simulink model "wb_try2"  (R2016b)
settings: Solver=FixedStepDiscrete  StartTime=0.0  StopTime=99/paramRadarMT.prf  RelTol=1e-3  EnableMultiTasking=on
PreLoadFcn:
  | helperslexMonostaticRadarMultipleTargetsParam()
undefined symbols (not defined in the file or in its folder): paramRadarMT, phased, physconst
libraries: phasedenvlib x5, phasedtxrxlib x4, phaseddetectlib x3, phasedwavlib x2, simulink x1, phasedbflib x1
CloseFcn:
  | clear paramRadarMT
Description:
  | Monostatic Radar with Three Targets
settings Model: Creator=The MathWorks, Inc.  LastModifiedBy=CHAITRA
settings DataIOCC: LimitDataPoints=on  SaveFormat=Array  SaveOutput=off  SaveTime=off
settings OptimizationCC: ExpressionDepthLimit=2147483647  LifeSpan=inf
settings DebuggingCC: ReadBeforeWriteMsg=DisableAll  WriteAfterWriteMsg=DisableAll  WriteAfterReadMsg=DisableAll  UnderspecifiedInitializationDetection=Classic  MergeDetectMultiDrivingBlocksExec=none  SolverPrmCheckMsg=warning  InheritedTsInSrcMsg=none  MultiTaskDSMMsg=none  FcnCallInpInsideContextMsg=warning  AllowSymbolicDim=off  StateNameClashWarn=warning  SFUnexpectedBacktrackingDiag=warning  SFNoUnconditionalDefaultTransitionDiag=warning  SFExecutionAtInitializationDiag=none
settings HardwareCC: ProdBitPerPointer=32  ProdBitPerSizeT=32  ProdBitPerPtrDiffT=32  ProdLargestAtomicFloat=None  ProdIntDivRoundTo=Undefined  ProdEndianess=Unspecified  ProdWordSize=32  ProdHWDeviceType=32-bit Generic
settings ModelReferenceCC: UpdateModelReferenceTargets=IfOutOfDate  PropagateSignalLabelsOutOfModel=off
settings SFSimCC: SFSimEcho=off  SimParseCustomCode=off
settings GRTTargetCC: TargetLangStandard=C89/C90 (ANSI)  GeneratePreprocessorConditionals=Disable all  CombineOutputUpdateFcns=off  GRTInterface=on
settings ConfigComp: CovMetricSettings=dw  CovHtmlReporting=on  CovSaveCumulativeToWorkspaceVar=on  CovSaveSingleToWorkspaceVar=on  CovExternalEMLEnable=off  CovSFcnEnable=off

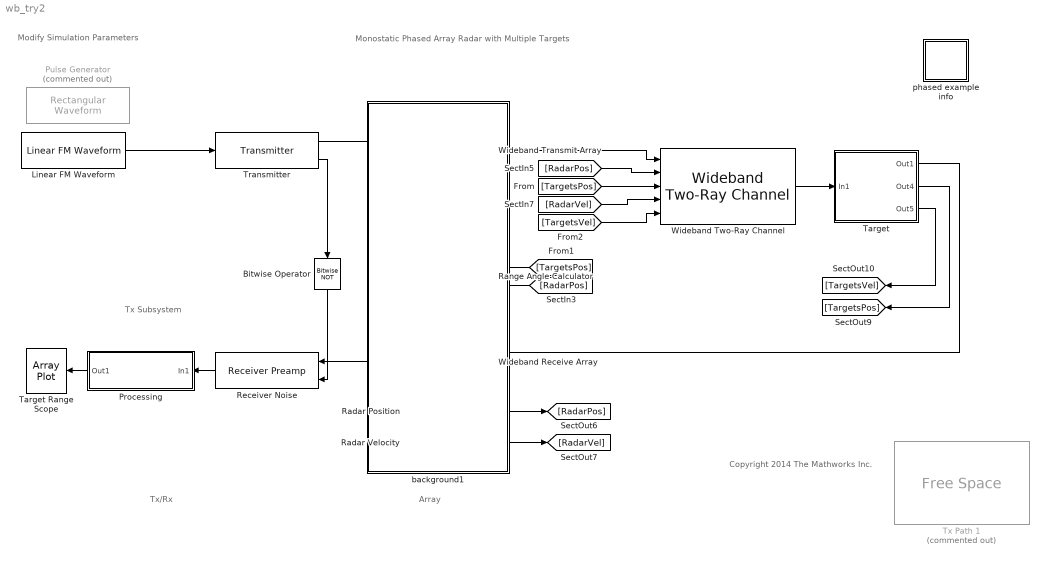
== system wb_try2 ==
  note: Monostatic Phased Array Radar with Multiple Targets
  note: Tx Subsystem
  note: Tx/Rx
  note: Modify Simulation Parameters
  note: Copyright 2014 The Mathworks Inc.
  note: Array
  Bitwise Operator : simulink/Logic and Bit Operations/Bitwise Operator  logicop=NOT  UseBitMask=off  BitMask=bin2dec('11011001')  BitMaskRealWorld=Stored Integer
  Linear FM Waveform : phasedwavlib/Linear FM Waveform  SampleRate=paramRadarMT.fs  DurationSpecification=Pulse width  PulseWidth=1/paramRadarMT.pulseBw  DutyCycle=0.5  PRF=paramRadarMT.prf  PRFSelectionInputPort=off  SweepBandwidth=1e5  SweepDirection=Up  SweepInterval=Positive  Envelope=Rectangular  OutputFormat=Pulses  NumSamples=100  NumPulses=1  SimulateUsing=Interpreted execution
  Processing : Subsystem
      mask Display: disp('Signal Processing')
  Pulse Generator : phasedwavlib/Rectangular Waveform  Commented=on  SampleRate=paramRadarMT.fs  DurationSpecification=Pulse width  PulseWidth=1/paramRadarMT.pulseBw  DutyCycle=0.5  PRF=paramRadarMT.prf  PRFSelectionInputPort=off  OutputFormat=Pulses  NumSamples=100  NumPulses=1  SimulateUsing=Interpreted execution
  Radar Position : Constant  Value=[ 0; 0; 0 ]  SampleTime=1/paramRadarMT.prf
  Radar Velocity : Constant  Value=[ 0; 0; 0 ]  SampleTime=1/paramRadarMT.prf
  Range Angle Calculator : phasedenvlib/Range Angle Calculator  Model=Free space  ReferencePositionSource=Input port  ReferencePosition=[ 0; 0; 0 ]  ReferenceAxesSource=Property  ReferenceAxes=eye( 3 )  Output=Angle  SimulateUsing=Interpreted execution
  Receiver Noise : phasedtxrxlib/Receiver Preamp  Gain=20  LossFactor=0  NoiseMethod=Noise temperature  NoiseFigure=0  ReferenceTemperature=290  SampleRateFromInputCheckbox=on  SampleRate=1e6  NoisePower=0  EnableInputPort=on  PhaseNoiseInputPort=off  SeedSource=Auto  Seed=0  SimulateUsing=Interpreted execution
  Target : Subsystem
      mask Display:
      | disp('Targets')
      | port_label('input',1,'X');
      | port_label('output',1,'Y');
      | port_label('output',2,'Pos');
      | port_label('output',3,'Vel');
  Target Range Scope : ArrayPlot
  Transmitter : phasedtxrxlib/Transmitter  PeakPower=paramRadarMT.peakPower/16  Gain=paramRadarMT.txGain  LossFactor=0  InUseOutputPort=on  CoherentOnTransmit=on  PhaseNoiseOutputPort=off  SeedSource=Auto  Seed=0  SimulateUsing=Interpreted execution
  Tx Path 1 : phasedenvlib/Free Space  Commented=on  PropagationSpeed=paramRadarMT.propSpeed  OperatingFrequency=paramRadarMT.fc  TwoWayPropagation=on  SampleRateFromInputCheckbox=on  SampleRate=1e6  MaximumDistanceSource=Property  MaximumDistance=10e3  MaximumNumInputSamplesSource=Auto  MaximumNumInputSamples=1000  SimulateUsing=Interpreted execution
  Wideband Receive Array : phasedtxrxlib/Wideband Receive Array  PropagationSpeed=paramRadarMT.propSpeed  SampleRateFromInputCheckbox=on  SampleRate=1e6  ModulatedInput=on  CarrierFrequency=paramRadarMT.fc  NumSubbands=64  Wavefront=Plane  EnablePolarization=off  WeightsInputPort=off  SimulateUsing=Interpreted execution  Sensor=phased.ULA('Element',phased.CosineAntennaElement(),'NumElements',4,'ElementSpacing',paramRadarMT.lambda/2)
  Wideband Transmit Array : phasedtxrxlib/Wideband Transmit Array  PropagationSpeed=paramRadarMT.propSpeed  SampleRateFromInputCheckbox=on  SampleRate=1e6  CarrierFrequency=paramRadarMT.fc  NumSubbands=64  EnablePolarization=off  WeightsInputPort=off  SimulateUsing=Interpreted execution  Sensor=phased.ULA('Element',phased.CosineAntennaElement(),'NumElements',4,'ElementSpacing',paramRadarMT.lambda/2)
  Wideband Two-Ray Channel : phasedenvlib/Wideband Two-Ray Channel  PropagationSpeed=physconst( 'LightSpeed' )  OperatingFrequency=paramRadarMT.fc  NumSubbands=64  SpecifyAtmosphere=off  Temperature=15  DryAirPressure=101325  WaterVapourDensity=7.5  LiquidWaterDensity=0  RainRate=0  SampleRateFromInputCheckbox=on  SampleRate=1e6  GroundReflectionCoefficient=-1  GroundRelativePermittivity=15  CombinedRaysOutput=on  MaximumDistanceSource=Property  MaximumDistance=500  MaximumNumInputSamplesSource=Auto  MaximumNumInputSamples=1000  SimulateUsing=Interpreted execution
  background1 : Subsystem  Description=Jammer
      mask Display: disp('')
  phased example info : Subsystem
      settings: OpenFcn=|
      | htmlpath = fullfile(matlabroot,'toolbox','phased','phaseddemos','html','slexMonostaticRadarExample.html');
      | web(htmlpath,'-helpbrowser');
      | clear htmlpath;
      mask Display: disp('Info')
  wires:
  Receiver Noise/1 -> Processing/1(In1)
  Processing/1(Out1) -> Target Range Scope/1
  Transmitter/1 -> Wideband Transmit Array/1
  Bitwise Operator/1 -> Receiver Noise/2
  Range Angle Calculator/1 -> Wideband Receive Array/2, Wideband Transmit Array/2
  [RadarPos] -> Range Angle Calculator/2
  Wideband Transmit Array/1 -> Wideband Two-Ray Channel/1
  [RadarVel] -> Wideband Two-Ray Channel/4
  [TargetsPos] -> Range Angle Calculator/1
  [TargetsVel] -> Wideband Two-Ray Channel/5
  [RadarPos] -> Wideband Two-Ray Channel/2
  Radar Velocity/1 -> [RadarVel]
  Radar Position/1 -> [RadarPos]
  Transmitter/2 -> Bitwise Operator/1
  [TargetsPos] -> Wideband Two-Ray Channel/3
  Target/2(Out4) -> [TargetsPos]
  Target/3(Out5) -> [TargetsVel]
  Target/1(Out1) -> Wideband Receive Array/1
  Wideband Receive Array/1 -> Receiver Noise/1
  Linear FM Waveform/1 -> Transmitter/1
  Wideband Two-Ray Channel/1 -> Target/1(In1)

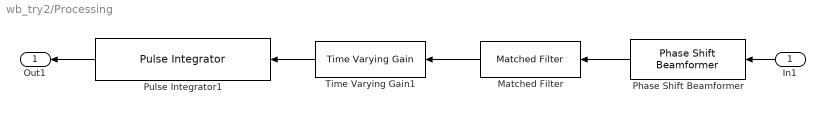
== system wb_try2/Processing ==
  In1 : Inport
  Matched Filter : phaseddetectlib/Matched Filter  CoefficientsSource=Property  Coefficients=paramRadarMT.matchingCoeff  SpectrumWindow=None  CustomSpectrumWindow=@hamming  SpectrumRange=[ 0, 1e5 ]  SampleRateFromInputCheckbox=on  SampleRate=1e6  SidelobeAttenuation=30  Beta=0.5  Nbar=4  GainOutputPort=off  MaximumNumInputSamplesSource=Auto  MaximumNumInputSamples=100  SimulateUsing=Interpreted execution
  Phase Shift Beamformer : phasedbflib/Phase Shift Beamformer  PropagationSpeed=paramRadarMT.propSpeed  OperatingFrequency=paramRadarMT.fc  DirectionSource=Property  Direction=[ 0; 0 ]  NumPhaseShifterBits=0  WeightsNormalization=Distortionless  WeightsOutputPort=off  SimulateUsing=Interpreted execution  SensorArray=phased.ULA('Element',phased.IsotropicAntennaElement(),'NumElements',4,'Taper',1,'ElementSpacing',paramRadarMT.lambda/2)
  Pulse Integrator1 : phaseddetectlib/Pulse Integrator  CoherentFlag=Noncoherent  N=10  V=0
  Time Varying Gain1 : phaseddetectlib/Time Varying Gain  RangeLossSource=Property  RangeLoss=paramRadarMT.rangeLoss  ReferenceLoss=paramRadarMT.referenceLoss  SimulateUsing=Interpreted execution
  Out1 : Outport
  wires:
  Time Varying Gain1/1 -> Pulse Integrator1/1
  Matched Filter/1 -> Time Varying Gain1/1
  Pulse Integrator1/1 -> Out1/1
  In1/1 -> Phase Shift Beamformer/1
  Phase Shift Beamformer/1 -> Matched Filter/1

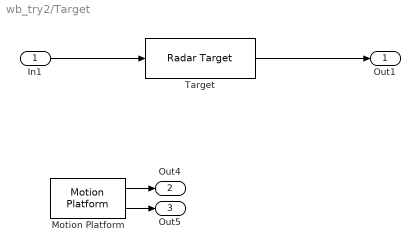
== system wb_try2/Target ==
  In1 : Inport
  Motion Platform : phasedenvlib/Motion Platform  MotionModel=Velocity  InitialPosition=paramRadarMT.targetPos  InitialVelocity=[ 0; 0; 0 ]  VelocitySource=Property  Velocity=paramRadarMT.targetVel  AccelerationSource=Property  Acceleration=[0;0;0]  InitialOrientationAxes=eye(3)  OrientationAxesOutputPort=off  ElapsedTimeSource=Auto  SampleRateFromInputCheckbox=on  SampleRate=1e6  SimulateUsing=Interpreted execution
  Target : phasedenvlib/Radar Target  EnablePolarization=off  Mode=Monostatic  MeanRCSSource=Property  ScatteringMatrixSource=Property  MeanRCS=paramRadarMT.targetRcs  ScatteringMatrix=eye( 2 )  Model=Nonfluctuating  PropagationSpeed=paramRadarMT.propSpeed  OperatingFrequency=paramRadarMT.fc  SeedSource=Auto  Seed=0  SimulateUsing=Interpreted execution
  Out1 : Outport
  Out4 : Outport  Port=2
  Out5 : Outport  Port=3
  wires:
  In1/1 -> Target/1
  Target/1 -> Out1/1
  Motion Platform/1 -> Out4/1
  Motion Platform/2 -> Out5/1

== system wb_try2/background1 ==

== system wb_try2/phased example info ==
